simulink library "commsdrhw_v2"  (Simulink 8.0)
settings: Solver=ode45  StartTime=0.0  StopTime=10.0  RelTol=1e-3
undefined symbols (not defined in the file or in its folder): sdruroot, setupsdru
settings Model: ForwardingTableString=||__slOldName__||commsdrhw_v2/USRP Receiver UHD||__slNewName__||commsdrhw_v2/SDRu Receiver||__slOldName__||commsdrhw_v2/USRP Receiver||__slNewName__||commsdrhw_v2/SDRu Receiver||__slOldName__||commsdrhw_v2/USRP Transmitter UHD||__slNewName__||commsdrhw_v2/SDRu Transmitter||__slOldName__||commsdrhw_v2/USRP Transmitter||__slNewName__||commsdrhw_v2/SDRu Transmitter  Creator=arogers  LastModifiedBy=esozer

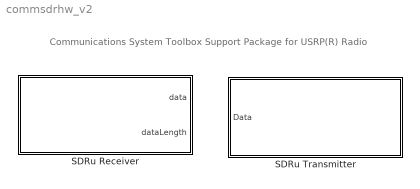
== system commsdrhw_v2 ==
  note: Communications System Toolbox Support Package for USRP(R) Radio
  SDRu Receiver : Subsystem  DialogController=usrpDDGCreate  DialogControllerArgs=DataTag0  LoadFcn=setupsdru(sdruroot, 'silent')  mask(SDRu Receiver){rxtx=rx, USRP2_IP='192.168.10.2', centerFrequency=2.45e9, centerFrequencySrc=Dialog, loOffset=0, loOffsetSrc=Dialog, gain=32, gainSrc=Dialog, decimInterp=512, decimInterpSrc=Dialog, USRP2_IP_NUM=[49 57 50 46 49 54 56 46 49 48 46 50], frameLength=362, outputDatatype=int16, overrunUnderrunPort=off, sampleTime=1, HOST_DATA_PORT=0, HOST_CONTROL_PORT=0, USRP2_DATA_PORT=0, USRP2_CONTROL_PORT=0, bufferMode=Continuous streaming, EnableBurstMode=off, NumFramesInBurst=100}
      mask prompts: rxtx "Rx or Tx block"; USRP2_IP "USRP IP Address"; centerFrequency "Center Frequency"; centerFrequencySrc "Center Frequency Src"; loOffset "LO Offset"; loOffsetSrc "LO Offset Src"; gainSrc "Gain Src"; decimInterp "Decimation Factor"; decimInterpSrc "Decimation Factor Src"; USRP2_IP_NUM "Numeric IP addr"; bufferMode "Buffer mode"; EnableBurstMode "Enable burst mode"; NumFramesInBurst "Number of frames in burst"
      mask help: Receive data from the Universal Software Radio Peripheral (USRP).
      mask init:
      | block = gcb;
      | blockH = gcbh;
      | maskDisplay = commblkusrp(block, 'maskDisplay');
      | commblkusrp(block, 'reconfigure');
      | commblkusrp(block, 'setDerivedParams');
      | % make sure do maskDisplay set_param after reconfiguring ports
      | set_param(blockH, 'maskDisplay', maskDisplay);
      mask Help: web(['file:///' sdruroot '/help/ref/sdrureceiver.html']);
      mask TypeOptions centerFrequencySrc: Dialog | Input port
      mask TypeOptions loOffsetSrc: Dialog | Input port
      mask TypeOptions gainSrc: Dialog | Input port
      mask TypeOptions decimInterpSrc: Dialog | Input port
      mask TypeOptions outputDatatype: int16 | double | single
      mask TypeOptions bufferMode: Continuous streaming | Guaranteed contiguous buffer | Guaranteed contiguous frame
      mask Display:
      | fprintf('SDRu\nReceiver');
      | port_label('output', 1, 'Data');
      | port_label('output', 2, 'Data Len');
  SDRu Transmitter : Subsystem  DialogController=usrpDDGCreate  DialogControllerArgs=DataTag1  LoadFcn=setupsdru(sdruroot, 'silent')  mask(SDRu Transmitter){rxtx=tx, USRP2_IP='192.168.10.2', centerFrequency=2.45e9, centerFrequencySrc=Dialog, loOffset=0, loOffsetSrc=Dialog, gain=8, gainSrc=Dialog, decimInterp=512, decimInterpSrc=Dialog, USRP2_IP_NUM=[49 57 50 46 49 54 56 46 49 48 46 50], frameLength=362, outputDatatype=int16, overrunUnderrunPort=off, sampleTime=1, dboardInfo=|, HOST_DATA_PORT=30000, HOST_CONTROL_PORT=30001, USRP2_DATA_PORT=32769, USRP2_CONTROL_PORT=32768, bufferMode=Continuous streaming, EnableBurstMode=off, NumFramesInBurst=100}
      mask dboardInfo=|
      | dbid: 0
      |           dbName: 'no db found'
      |          freqMin: 0
      |          freqMax: 0
      |          gainMin: 0
      |          gainMax: 0
      |     gainStepSize: 0
      mask prompts: rxtx "Rx or Tx block"; USRP2_IP "USRP IP Address"; centerFrequency "Center Frequency"; centerFrequencySrc "Center Frequency Src"; loOffset "LO Offset"; loOffsetSrc "LO Offset Src"; gainSrc "Gain Src"; decimInterp "Interpolation Factor"; decimInterpSrc "Interpolation Src"; USRP2_IP_NUM "Numeric IP addr"; frameLength "Frame Length"; dboardInfo "Daughterboard Info"; HOST_DATA_PORT "Host Data Port"; HOST_CONTROL_PORT "Host Control Port"; USRP2_DATA_PORT "USRP2 Data Port"; USRP2_CONTROL_PORT "USRP2 Control Port"; bufferMode "Buffer mode"; EnableBurstMode "Enable burst mode"; NumFramesInBurst "Number of frames in burst"
      mask help: Send data to the Universal Software Radio Peripheral (USRP).
      mask init:
      | block = gcb;
      | blockH = gcbh;
      | maskDisplay = commblkusrp(block, 'maskDisplay');
      | commblkusrp(block, 'reconfigure');
      | commblkusrp(block, 'setDerivedParams');
      | % make sure do maskDisplay set_param after reconfiguring ports
      | set_param(blockH, 'maskDisplay', maskDisplay);
      mask Help: web(['file:///' sdruroot '/help/ref/sdrutransmitter.html']);
      mask TypeOptions centerFrequencySrc: Dialog | Input port
      mask TypeOptions loOffsetSrc: Dialog | Input port
      mask TypeOptions gainSrc: Dialog | Input port
      mask TypeOptions decimInterpSrc: Dialog | Input port
      mask TypeOptions outputDatatype: int16 | double | single
      mask TypeOptions bufferMode: Continuous streaming | Guaranteed contiguous buffer | Guaranteed contiguous frame
      mask Display:
      | fprintf('SDRu\nTransmitter');
      | port_label('input', 1, 'Data');

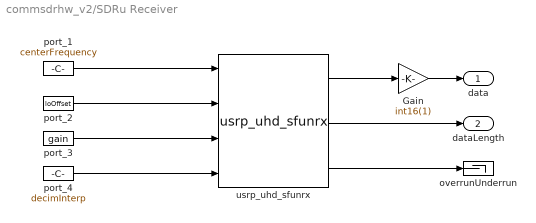
== system commsdrhw_v2/SDRu Receiver ==
  Gain : Gain  Gain=int16(1)  ParamDataTypeStr=Inherit: Inherit from 'Gain'  OutDataTypeStr=int16
  overrunUnderrun : Terminator
  port_1 : Constant  Value=centerFrequency
  port_2 : Constant  Value=loOffset
  port_3 : Constant  Value=gain
  port_4 : Constant  Value=decimInterp
  usrp_uhd_sfunrx : S-Function  FunctionName=usrp_uhd_sfunrx  Parameters=IPAddrAsInt8Array, BoardId, SParameter3, DportDtype, BuffMode, SParameter6, SampleTime  EnableBusSupport=off  mask(usrp_uhd_sfunrx){SFunctionSpec=void simRecvData_c(  int32  work4, double u1, double u2, double u3, double u4, uint32 p3, capi_DataportDatatypeEnumT p4, complex<int16> y1[p3], uint32 y2[1], uint32 y3[1], capi_UsrpErrStatEnumT work2[1], int8 work3[1024]), SParameter1=USRP2_IP, SParameter2=rxtx, SParameter3=frameLength, SParameter4=outputDatatype, SParameter5=bufferMode, SParameter6=NumFramesInBurst, SampleTime=sampleTime, ShowSpec=off}
      mask prompts: SParameter1 "P1:"; SParameter2 "P2:"; SParameter3 "P3:"; SParameter4 "P4:"; SParameter5 "P5:"; SParameter6 "P6:"; SampleTime "Sample time (-1 for inherited):"; ShowSpec "Display function specification"
      mask help: usrp_uhd_sfunrx
      mask init:
      | IPAddrAsInt8Array = [int8(SParameter1), 0];
      | switch (SParameter2)
      |     case 'rx', BoardId = BoardIdSLCapiEnumT.RxId;
      |     case 'tx', BoardId = BoardIdSLCapiEnumT.TxId;
      |     otherwise, BoardId = BoardIdSLCapiEnumT.RxId;
      | end
      | switch (SParameter4)
      |     case 'int16',  DportDtype = DataPortDataTypeSLCapiEnumT.DPortDTypeCInt16;
      |     case 'single', DportDtype = DataPortDataTypeSLCapiEnumT.DPortDTypeCSingle;
      |     case 'double', DportDtype = DataPortDataTypeSLCapiEnumT.DPortDTypeCDouble;
      |     otherwise,     DportDtype = DataPortDataTypeSLCapiEnumT.DPortDTypeCInt16;            
      | end
      | switch (SParameter5)
      |     case 'Continuous streaming',         BuffMode = BufferModeSLCapiEnumT.BuffModeContinuous;
      |     case 'Guaranteed contiguous buffer', BuffMode = BufferModeSLCapiEnumT.BuffModeContigBuff;
      |     case 'Guaranteed contiguous frame',  BuffMode = BufferModeSLCapiEnumT.BuffModeContigFrame;
      |     otherwise,                           BuffMode = BufferModeSLCapiEnumT.BuffModeContinuous;
      | end
      mask Help: usrp_uhd_sfunrx
      mask Callback ShowSpec:
      | if strcmp(get_param(gcbh, 'ShowSpec'), 'on')
      |   set_param(gcbh, 'MaskDisplay', sprintf('fprintf(''%s'');', get_param(gcbh, 'SFunctionSpec')));
      | else
      |   set_param(gcbh, 'MaskDisplay', sprintf('fprintf(''%s'');', get_param(gcbh, 'FunctionName')));
      | end
      mask Display: fprintf('usrp_uhd_sfunrx');
  data : Outport
  dataLength : Outport  Port=2
  wires:
  usrp_uhd_sfunrx/1 -> Gain/1
  port_1/1 -> usrp_uhd_sfunrx/1
  port_3/1 -> usrp_uhd_sfunrx/3
  port_4/1 -> usrp_uhd_sfunrx/4
  usrp_uhd_sfunrx/3 -> overrunUnderrun/1
  usrp_uhd_sfunrx/2 -> dataLength/1
  Gain/1 -> data/1
  port_2/1 -> usrp_uhd_sfunrx/2

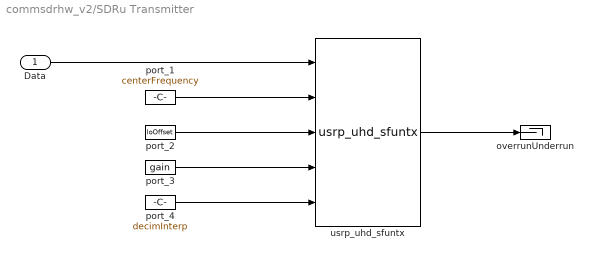
== system commsdrhw_v2/SDRu Transmitter ==
  Data : Inport
  overrunUnderrun : Terminator
  port_1 : Constant  Value=centerFrequency
  port_2 : Constant  Value=loOffset
  port_3 : Constant  Value=gain
  port_4 : Constant  Value=decimInterp
  usrp_uhd_sfuntx : S-Function  FunctionName=usrp_uhd_sfuntx  Parameters=IPAddrAsInt8Array, BoardId, SParameter3, DportDtype, BuffMode, SParameter6  EnableBusSupport=off  mask(usrp_uhd_sfuntx){SFunctionSpec=void simSendData_c(  int32  work4, complex<int16> u1[], double u2, double u3, double u4, double u5, uint32 work5, capi_DataportDatatypeEnumT work6, uint32 y1[1], capi_UsrpErrStatEnumT work2[1], int8 work3[1024]), SParameter1=USRP2_IP, SParameter2=rxtx, SParameter3=frameLength, SParameter4=outputDatatype, SParameter5=bufferMode, SParameter6=NumFramesInBurst, ShowSpec=off}
      mask prompts: SParameter1 "P1:"; SParameter2 "P2:"; SParameter3 "P3:"; SParameter4 "P4:"; SParameter5 "P5:"; SParameter6 "P6:"; ShowSpec "Display function specification"
      mask help: usrp_uhd_sfuntx
      mask init:
      | IPAddrAsInt8Array = [int8(SParameter1), 0];
      | switch (SParameter2)
      |     case 'rx', BoardId = BoardIdSLCapiEnumT.RxId;
      |     case 'tx', BoardId = BoardIdSLCapiEnumT.TxId;
      |     otherwise, BoardId = BoardIdSLCapiEnumT.RxId;
      | end
      | switch (SParameter4)
      |     otherwise,     DportDtype = DataPortDataTypeSLCapiEnumT.DPortDTypeCInt16;            
      | end
      | switch (SParameter5)
      |     case 'Continuous streaming',         BuffMode = BufferModeSLCapiEnumT.BuffModeContinuous;
      |     case 'Guaranteed contiguous buffer', BuffMode = BufferModeSLCapiEnumT.BuffModeContigBuff;
      |     case 'Guaranteed contiguous frame',  BuffMode = BufferModeSLCapiEnumT.BuffModeContigFrame;
      |     otherwise,                           BuffMode = BufferModeSLCapiEnumT.BuffModeContinuous;
      | end
      mask Help: usrp_uhd_sfuntx
      mask Callback ShowSpec:
      | if strcmp(get_param(gcbh, 'ShowSpec'), 'on')
      |   set_param(gcbh, 'MaskDisplay', sprintf('fprintf(''%s'');', get_param(gcbh, 'SFunctionSpec')));
      | else
      |   set_param(gcbh, 'MaskDisplay', sprintf('fprintf(''%s'');', get_param(gcbh, 'FunctionName')));
      | end
      mask Display: fprintf('usrp_uhd_sfuntx');
  wires:
  Data/1 -> usrp_uhd_sfuntx/1
  port_1/1 -> usrp_uhd_sfuntx/2
  port_3/1 -> usrp_uhd_sfuntx/4
  port_4/1 -> usrp_uhd_sfuntx/5
  usrp_uhd_sfuntx/1 -> overrunUnderrun/1
  port_2/1 -> usrp_uhd_sfuntx/3
